simulink model "regs_12B"  (R2018a)
settings: Solver=ode3  StartTime=0.0  StopTime=10.0  FixedStep=.01  RelTol=1e-3  EnableMultiTasking=on
model workspace (MAT data in the model file):
  F = [47.5030304796; 46.9110614304; 47.028984707; 45.6862216169; 44.6182372756; 0]
  FR = [-46.5418915863 -46.5418915863 -46.5418915863 -46.5418915863 -46.5418915863 -46.5418915863 -46.5418915863 -46.5418915863 -46.5418915863 -46.5418915863 -46.5418915863 -46.5418915863 ... (901 elements, 1x901)]
  InputSize = 6
  M = [13.6965475483 27.5033300826 -29.1231309962 -36.2545983973 -28.5352204611 23.5897220685 -14.907640199 1.71607773467 -6.59423100681 35.1253819893 -6.10963272822 7.71481328081 ... (3003 elements, 1001x3)]
  N = 24
  T = table
  T.data = {[13.6965475483 27.5033300826 -29.1231309962 -36.2545983973 -28.5352204611 23.5897220685 -14.907640199 1.71607773467 -6.59423100681 35.1253819893 -6.10963272822 7.71481328081 ... (1001 elements, 1001x1)], [-4.50869960006 8.78080542631 13.3775275088 31.9867982316 4.18537435026 16.5092867395 24.6932352308 2.38519814211 8.8890132209 -4.02964212249 -4.46675798218 1.79304742838 ... (1001 elements, 1001x1)], [-31.9718041188 -26.9402342951 13.2152788717 -38.0977072288 -36.3083467361 23.117797395 10.5331769063 33.1487702757 -5.61173456269 9.59308730026 21.4490888958 -5.45903036842 ... (1001 elements, 1001x1)]}
  T.ndims = 2
  T.nrows = 1001
  T.nvars = 3
  T.varnames = {'Var1', 'Var2', 'Var3'}
  T.props.versionSavedFrom = 2.2
  T.props.minCompatibleVersion = 1
  T.props.incompatibilityMsg = ''
  T.props.VersionSavedFrom = 2.2
  T.props.Description = ''
  T.props.DimensionNames = {'Row', 'Variables'}
  T.props.UserData = []
  T.props.VariableDescriptions = {}
  T.props.VariableUnits = {}
  T.props.VariableContinuity = {}
  X = [0.032483647429 0.400056291337 1.71698946504 0.13508020958 0.621497120838 1.65324546556 1.22373682905 1.82920074721 1.76822087632 0.490626067878 1.91640381392 0.904593399727 1.77711628782 0.929700787381 1.1704427226 0.0233580241983 1.45687078118 0.830600702987 0.237274970231 1.19251283181 0.00937571906531 1.87890955837 1.38282407714 0.543596154356 1.5074746628 1.31666384939 0.567420251723 1.07122901547 0.120432144233 1.35485454959 1.84576620576 0.933277353969]
  a1 = -5.99281334265
  a2 = 6.7586120696
  a3 = -8.48382923723
  axial = 0
  axial_change = [-31.4255261802 -30.7695758416 -31.1885211647 -29.9884626265 -30.6698057294 -31.9546590717 -31.9773114122 -31.0590125801 -31.4973929014 -31.4591407909 -31.9452553476 -31.5912458676 ... (1000 elements, 1000x1)]
  cmd.dt = 0.01
  cmd.transition_v = [0 50 90 1000]
  cmd.transition_y = [0 0 1 1]
  cs : Simulink.ConfigSet (value not decoded)
  curPath = '/Users/khouloud.gaaloul/Documents/Projects/QRA-LocalSearch/Local Search Algorithms/Problems'
  d = 33
  hcvdt_cmd_fcs_dps2 = [0 0 0 0 0 0 0 0 0 0 0 0 ... (1000 elements, 1000x1)]
  height = 0
  height_change = [-31.99975 -31.8 -31.8 -31.8 -31.99975 -31.8 -31.8 -31.8 -31.99975 -31.8 -31.99975 -31.8 ... (1000 elements, 1000x1)]
  hws = Simulink.ModelWorkspace
  i = 7
  j = 16
  lcvdt_cmd_fcs_dps2 = [-172.441967394 -126.914225002 101.408793207 185.523827088 35.8854623366 -8.64188069371 100.038910088 117.411213524 -22.955981386 -181.02871483 29.1905053694 73.1255676915 ... (1000 elements, 1000x1)]
  list(1).name = 'F'
  list(1).size = [6 1]
  list(1).bytes = 48
  list(1).class = 'double'
  list(1).global = 0
  list(1).sparse = 0
  list(1).complex = 0
  list(1).nesting.function = 'simreg'
  list(1).nesting.level = 1
  list(1).persistent = 0
  list(2).name = 'FR'
  list(2).size = [1 901]
  list(2).bytes = 7208
  list(2).class = 'double'
  list(2).global = 0
  list(2).sparse = 0
  list(2).complex = 0
  list(2).nesting.function = 'simreg'
  list(2).nesting.level = 1
  list(2).persistent = 0
  list(3).name = 'InputSize'
  list(3).size = [1 1]
  list(3).bytes = 8
  list(3).class = 'double'
  list(3).global = 0
  list(3).sparse = 0
  list(3).complex = 0
  list(3).nesting.function = 'simreg'
  list(3).nesting.level = 1
  list(3).persistent = 0
  list(4).name = 'N'
  list(4).size = [1 1]
  list(4).bytes = 8
  list(4).class = 'double'
  list(4).global = 0
  list(4).sparse = 0
  list(4).complex = 0
  list(4).nesting.function = 'simreg'
  list(4).nesting.level = 1
  list(4).persistent = 0
  list(5).name = 'X'
  list(5).size = [6 2002]
  list(5).bytes = 96096
  list(5).class = 'double'
  list(5).global = 0
  list(5).sparse = 0
  list(5).complex = 0
  list(5).nesting.function = 'simreg'
  list(5).nesting.level = 1
  list(5).persistent = 0
  list(6).name = 'curPath'
  list(6).size = [1 78]
  list(6).bytes = 156
  list(6).class = 'char'
  list(6).global = 0
  list(6).sparse = 0
  list(6).complex = 0
  list(6).nesting.function = 'simreg'
  list(6).nesting.level = 1
  list(6).persistent = 0
  list(7).name = 'd'
  list(7).size = [1 1]
  list(7).bytes = 8
  list(7).class = 'double'
  list(7).global = 0
  list(7).sparse = 0
  list(7).complex = 0
  list(7).nesting.function = 'simreg'
  list(7).nesting.level = 1
  list(7).persistent = 0
  list(8).name = 'hcvdt_cmd_fcs_dps2'
  list(8).size = [1000 1]
  list(8).bytes = 8000
  list(8).class = 'double'
  list(8).global = 0
  list(8).sparse = 0
  list(8).complex = 0
  list(8).nesting.function = 'simreg'
  list(8).nesting.level = 1
  list(8).persistent = 0
  list(9).name = 'hws'
  list(9).size = [1 1]
  list(9).bytes = 0
  list(9).class = 'Simulink.ModelWorkspace'
  list(9).global = 0
  list(9).sparse = 0
  list(9).complex = 0
  list(9).nesting.function = 'simreg'
  list(9).nesting.level = 1
  list(9).persistent = 0
  list(10).name = 'i'
  list(10).size = [1 1]
  list(10).bytes = 8
  list(10).class = 'double'
  list(10).global = 0
  list(10).sparse = 0
  list(10).complex = 0
  list(10).nesting.function = 'simreg'
  list(10).nesting.level = 1
  list(10).persistent = 0
  list(11).name = 'j'
  list(11).size = [1 1]
  list(11).bytes = 8
  list(11).class = 'double'
  list(11).global = 0
  list(11).sparse = 0
  list(11).complex = 0
  list(11).nesting.function = 'simreg'
  list(11).nesting.level = 1
  list(11).persistent = 0
  list(12).name = 'lcvdt_cmd_fcs_dps2'
  list(12).size = [1000 1]
  list(12).bytes = 8000
  list(12).class = 'double'
  list(12).global = 0
  list(12).sparse = 0
  list(12).complex = 0
  list(12).nesting.function = 'simreg'
  list(12).nesting.level = 1
  list(12).persistent = 0
  list(13).name = 'list'
  list(13).size = [24 1]
  list(13).bytes = 35056
  list(13).class = 'struct'
  list(13).global = 0
  list(13).sparse = 0
  list(13).complex = 0
  list(13).nesting.function = 'simreg'
  list(13).nesting.level = 1
  list(13).persistent = 0
  list(14).name = 'mcvdt_cmd_fcs_dps2'
  list(14).size = [1000 1]
  list(14).bytes = 8000
  list(14).class = 'double'
  list(14).global = 0
  list(14).sparse = 0
  list(14).complex = 0
  list(14).nesting.function = 'simreg'
  list(14).nesting.level = 1
  list(14).persistent = 0
  list(15).name = 'modelpath'
  list(15).size = [1 82]
  list(15).bytes = 164
  list(15).class = 'char'
  list(15).global = 0
  list(15).sparse = 0
  list(15).complex = 0
  list(15).nesting.function = 'simreg'
  list(15).nesting.level = 1
  list(15).persistent = 0
  list(16).name = 'n'
  list(16).size = [1 1]
  list(16).bytes = 8
  list(16).class = 'double'
  list(16).global = 0
  list(16).sparse = 0
  list(16).complex = 0
  list(16).nesting.function = 'simreg'
  list(16).nesting.level = 1
  list(16).persistent = 0
  list(17).name = 'nbrInputs'
  list(17).size = [1 1]
  list(17).bytes = 8
  list(17).class = 'double'
  list(17).global = 0
  list(17).sparse = 0
  list(17).complex = 0
  list(17).nesting.function = 'simreg'
  list(17).nesting.level = 1
  list(17).persistent = 0
  list(18).name = 'nbrTimeSteps'
  list(18).size = [1 1]
  list(18).bytes = 8
  list(18).class = 'double'
  list(18).global = 0
  list(18).sparse = 0
  list(18).complex = 0
  list(18).nesting.function = 'simreg'
  list(18).nesting.level = 1
  list(18).persistent = 0
  list(19).name = 'ncvdt_cmd_fcs_dps2'
  list(19).size = [1000 1]
  list(19).bytes = 8000
  list(19).class = 'double'
  list(19).global = 0
  list(19).sparse = 0
  list(19).complex = 0
  list(19).nesting.function = 'simreg'
  list(19).nesting.level = 1
  list(19).persistent = 0
  list(20).name = 'simOut'
  list(20).size = [1 1]
  list(20).bytes = 54442
  list(20).class = 'Simulink.SimulationOutput'
  list(20).global = 0
  list(20).sparse = 0
  list(20).complex = 0
  list(20).nesting.function = 'simreg'
  list(20).nesting.level = 1
  list(20).persistent = 0
  list(21).name = 't'
  list(21).size = [1 1]
  list(21).bytes = 8
  list(21).class = 'double'
  list(21).global = 0
  list(21).sparse = 0
  list(21).complex = 0
  list(21).nesting.function = 'simreg'
  list(21).nesting.level = 1
  list(21).persistent = 0
  list(22).name = 'var'
  list(22).size = [1 1]
  list(22).bytes = 140328
  list(22).class = 'struct'
  list(22).global = 0
  list(22).sparse = 0
  list(22).complex = 0
  list(22).nesting.function = 'simreg'
  list(22).nesting.level = 1
  list(22).persistent = 0
  list(23).name = 'varout'
  list(23).size = [1000 5]
  list(23).bytes = 40000
  list(23).class = 'double'
  list(23).global = 0
  list(23).sparse = 0
  list(23).complex = 0
  list(23).nesting.function = 'simreg'
  list(23).nesting.level = 1
  list(23).persistent = 0
  list(24).name = 'xcvdt_cmd_fcs_dps2'
  list(24).size = [1000 1]
  list(24).bytes = 8000
  list(24).class = 'double'
  list(24).global = 0
  list(24).sparse = 0
  list(24).complex = 0
  list(24).nesting.function = 'simreg'
  list(24).nesting.level = 1
  list(24).persistent = 0
  mcvdt_cmd_fcs_dps2 = [0 0 0 0 0 0 0 0 0 0 0 0 ... (1000 elements, 1000x1)]
  model_cs : Simulink.ConfigSet (value not decoded)
  modelpath = '/Users/khouloud.gaaloul/Documents/Projects/QRA-LocalSearch/Simulink Models/3_regulators/'
  n = 6
  nbrInputs = 16
  nbrTimeSteps = 1001
  ncvdt_cmd_fcs_dps2 = [0 0 0 0 0 0 0 0 0 0 0 0 ... (1000 elements, 1000x1)]
  pitch = 0
  pitch_change = [-29.1847957495 -33.8637964543 -47.1499761463 -47.1433778125 -41.276337879 -45.6028204159 -37.5507526458 -39.9406146771 -31.3489497461 -28.9458637417 -26.1569554928 -41.8886302088 ... (1000 elements, 1000x1)]
  req = 'R10'
  roll = 0
  roll_change = [-41.4686910833 -44.5265370434 -48.3240218587 -45.9838380142 -45.0248995082 -48.7661309065 -46.4562699575 -48.9496331544 -43.3304519808 -46.1818460958 -48.131234837 -44.5028232735 ... (1000 elements, 1000x1)]
  simOut = Simulink.SimulationOutput
  simOut.Data.tout = [0.01 0.02 0.03 0.04 0.05 0.06 0.07 0.08 0.09 0.1 0.11 0.12 ... (1000 elements, 1000x1)]
  simOut.Data.varout = [-172.441967394 -126.914225002 101.408793207 185.523827088 35.8854623366 -8.64188069371 100.038910088 117.411213524 -22.955981386 -181.02871483 29.1905053694 73.1255676915 ... (5000 elements, 1000x5)]
  simOut.Metadata = Simulink.SimulationMetadata
  simOut.Metadata.ModelInfo.ModelName = 'regs'
  simOut.Metadata.ModelInfo.ModelVersion = '1.40'
  simOut.Metadata.ModelInfo.ModelFilePath = '/Users/khouloud.gaaloul/Documents/Projects/QRA-Search/SimulinkModels/3_regulators/regs.slx'
  simOut.Metadata.ModelInfo.UserID = 'khouloud.gaaloul'
  simOut.Metadata.ModelInfo.MachineName = ''
  simOut.Metadata.ModelInfo.Platform = 'MACI64'
  simOut.Metadata.ModelInfo.ModelStructuralChecksum = [173027761; 2281278173; 3875996436; 2760024160]
  simOut.Metadata.ModelInfo.SimulationMode = 'normal'
  simOut.Metadata.ModelInfo.StartTime = 0
  simOut.Metadata.ModelInfo.StopTime = 10
  simOut.Metadata.ModelInfo.SolverInfo.Type = 'Fixed-Step'
  simOut.Metadata.ModelInfo.SolverInfo.Solver = 'FixedStepDiscrete'
  simOut.Metadata.ModelInfo.SolverInfo.FixedStepSize = 0.01
  simOut.Metadata.ModelInfo.SimulinkVersion.Name = 'Simulink'
  simOut.Metadata.ModelInfo.SimulinkVersion.Version = '8.7'
  simOut.Metadata.ModelInfo.SimulinkVersion.Release = '(R2016a)'
  simOut.Metadata.ModelInfo.SimulinkVersion.Date = '10-Feb-2016'
  simOut.Metadata.TimingInfo.WallClockTimestampStart = '2018-03-19 12:10:18.328231'
  simOut.Metadata.TimingInfo.WallClockTimestampStop = '2018-03-19 12:10:19.216989'
  simOut.Metadata.TimingInfo.InitializationElapsedWallTime = 0.857562
  simOut.Metadata.TimingInfo.ExecutionElapsedWallTime = 0.0059
  simOut.Metadata.TimingInfo.TerminationElapsedWallTime = 0.025314
  simOut.Metadata.TimingInfo.TotalElapsedWallTime = 0.888776
  simOut.Metadata.ExecutionInfo.StopEvent = 'ReachedStopTime'
  simOut.Metadata.ExecutionInfo.StopEventSource = []
  simOut.Metadata.ExecutionInfo.StopEventDescription = 'Reached stop time of 10'
  simOut.Metadata.ExecutionInfo.ErrorDiagnostic = []
  simOut.Metadata.ExecutionInfo.WarningDiagnostics = struct([])
  simOut.Metadata.AppInfo = struct()
  t = [0 0.01 0.02 0.03 0.04 0.05 0.06 0.07 0.08 0.09 0.1 0.11 ... (1001 elements, 1001x1)]
  u = [0.032483647429 0.032483647429 0.032483647429 0.032483647429 0.032483647429 0.032483647429 0.032483647429 0.032483647429 0.032483647429 0.032483647429 0.032483647429 0.032483647429 ... (16016 elements, 1001x16)]
  var.time = [0 0.01 0.02 0.03 0.04 0.05 0.06 0.07 0.08 0.09 0.1 0.11 ... (1001 elements, 1x1001)]
  var.signals(1).values = [0 0 0 0 0 0 0 0 0 0 0 0 ... (1001 elements, 1001x1)]
  var.signals(1).dimensions = 1
  var.signals(2).values = [0 0 0 0 0 0 0 0 0 0 0 0 ... (1001 elements, 1001x1)]
  var.signals(2).dimensions = 1
  var.signals(3).values = [-32.7185675438 -18.5522849548 3.78001601081 15.5815188083 36.1819132054 -17.2231806876 -17.5943876227 -13.0057864031 9.37261247594 -32.1369418892 10.1264127632 10.0220220005 ... (1001 elements, 1001x1)]
  var.signals(3).dimensions = 1
  var.signals(4).values = [0 0 0 0 0 0 0 0 0 0 0 0 ... (1001 elements, 1001x1)]
  var.signals(4).dimensions = 1
  var.signals(5).values = [0 0 0 0 0 0 0 0 0 0 0 0 ... (1001 elements, 1001x1)]
  var.signals(5).dimensions = 1
  var.signals(6).values = [0 0 0 0 0 0 0 0 0 0 0 0 ... (1001 elements, 1001x1)]
  var.signals(6).dimensions = 1
  var.signals(7).values = [0 0 0 0 0 0 0 0 0 0 0 0 ... (1001 elements, 1001x1)]
  var.signals(7).dimensions = 1
  var.signals(8).values = [0 0 0 0 0 0 0 0 0 0 0 0 ... (1001 elements, 1001x1)]
  var.signals(8).dimensions = 1
  var.signals(9).values = [0 0 0 0 0 0 0 0 0 0 0 0 ... (1001 elements, 1001x1)]
  var.signals(9).dimensions = 1
  var.signals(10).values = [0 0 0 0 0 0 0 0 0 0 0 0 ... (1001 elements, 1001x1)]
  var.signals(10).dimensions = 1
  var.signals(11).values = [-29.3225790184 21.8891959243 -11.8121125634 -28.6095603327 30.5189783332 -22.8969150265 17.132242283 30.9103401859 -35.8426218327 -15.1947880413 -18.4250967621 -31.7844478779 ... (1001 elements, 1001x1)]
  var.signals(11).dimensions = 1
  var.signals(12).values = [0 0 0 0 0 0 0 0 0 0 0 0 ... (1001 elements, 1001x1)]
  var.signals(12).dimensions = 1
  var.signals(13).values = [0 0 0 0 0 0 0 0 0 0 0 0 ... (1001 elements, 1001x1)]
  var.signals(13).dimensions = 1
  var.signals(14).values = [0 0 0 0 0 0 0 0 0 0 0 0 ... (1001 elements, 1001x1)]
  var.signals(14).dimensions = 1
  var.signals(15).values = [0 0 0 0 0 0 0 0 0 0 0 0 ... (1001 elements, 1001x1)]
  var.signals(15).dimensions = 1
  var.signals(16).values = [0 0 0 0 0 0 0 0 0 0 0 0 ... (1001 elements, 1001x1)]
  var.signals(16).dimensions = 1
  varout = [-172.441967394 -126.914225002 101.408793207 185.523827088 35.8854623366 -8.64188069371 100.038910088 117.411213524 -22.955981386 -181.02871483 29.1905053694 73.1255676915 ... (5000 elements, 1000x5)]
  vars = {'dt'; 'transition_v'; 'transition_y'}
  xcvdt_cmd_fcs_dps2 = [0 0 0 0 0 0 0 0 0 0 0 0 ... (1000 elements, 1000x1)]
  yaw = 0
  yaw_change = [-49.1533965478 -48.6929062567 -47.6689253182 -47.3940427916 -49.3847503901 -46.8626914945 -44.1531478971 -48.0156975418 -49.8912914581 -49.5126245185 -48.3496741118 -48.8753270352 ... (1000 elements, 1000x1)]
undefined symbols (not defined in the file): dt, transition_v, transition_y
libraries: simulink x2
(part 1 of 2)
settings Model: Creator=elliocm  LastModifiedBy=khouloud.gaaloul
settings DataIOCC: ExternalInput=[t,u]  LimitDataPoints=on  LoadExternalInput=on  SaveFormat=Array  SignalLoggingSaveFormat=ModelDataLogs
settings OptimizationCC: ExpressionDepthLimit=2147483647  LifeSpan=inf
settings DebuggingCC: UnderspecifiedInitializationDetection=Classic  MergeDetectMultiDrivingBlocksExec=none  SolverPrmCheckMsg=warning  FcnCallInpInsideContextMsg=warning  StateNameClashWarn=warning  SFUnexpectedBacktrackingDiag=warning  SFNoUnconditionalDefaultTransitionDiag=warning  SFExecutionAtInitializationDiag=none
settings HardwareCC: ProdBitPerPointer=32  ProdBitPerSizeT=32  ProdBitPerPtrDiffT=32  ProdLargestAtomicFloat=None  ProdIntDivRoundTo=Undefined  ProdEndianess=Unspecified  ProdWordSize=32  ProdHWDeviceType=32-bit Generic
settings ModelReferenceCC: PropagateSignalLabelsOutOfModel=off
settings CodeAppCC: StateflowObjectComments=on
settings GRTTargetCC: TargetLangStandard=C89/C90 (ANSI)  GeneratePreprocessorConditionals=Disable all  CombineOutputUpdateFcns=off  GRTInterface=on
settings ConfigComp: CovMetricSettings=dw  CovHtmlReporting=on  CovSaveCumulativeToWorkspaceVar=on  CovSaveSingleToWorkspaceVar=on  CovExternalEMLEnable=off

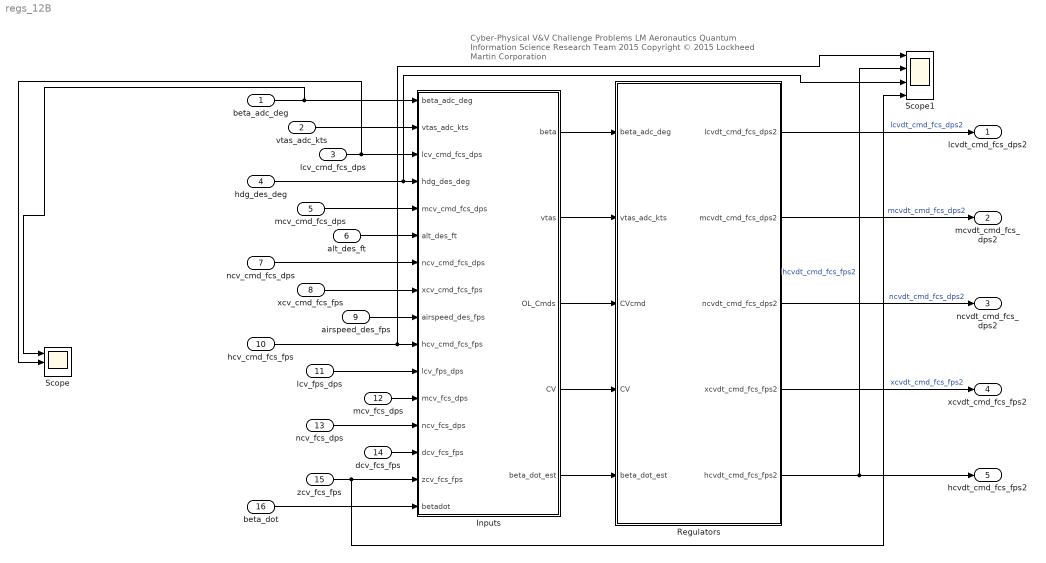
== system regs_12B ==
  note: Cyber-Physical V&V Challenge Problems
      | LM Aeronautics Quantum Information Science Research Team 2015
      | Copyright © 2015 Lockheed Martin Corporation
  beta_adc_deg : Inport  OutDataTypeStr=double
  vtas_adc_kts : Inport  Port=2  OutDataTypeStr=double
  "lcv_cmd_fcs_dps " : Inport  Port=3  OutDataTypeStr=double
  hdg_des_deg : Inport  Port=4  OutDataTypeStr=double
  mcv_cmd_fcs_dps : Inport  Port=5  OutDataTypeStr=double
  alt_des_ft : Inport  Port=6  OutDataTypeStr=double
  ncv_cmd_fcs_dps : Inport  Port=7  OutDataTypeStr=double
  xcv_cmd_fcs_fps : Inport  Port=8  OutDataTypeStr=double
  airspeed_des_fps : Inport  Port=9  OutDataTypeStr=double
  hcv_cmd_fcs_fps : Inport  Port=10  OutDataTypeStr=double
  lcv_fps_dps : Inport  Port=11  OutDataTypeStr=double
  mcv_fcs_dps : Inport  Port=12  OutDataTypeStr=double
  ncv_fcs_dps : Inport  Port=13  OutDataTypeStr=double
  dcv_fcs_fps : Inport  Port=14  OutDataTypeStr=double
  zcv_fcs_fps : Inport  Port=15  OutDataTypeStr=double
  beta_dot : Inport  Port=16  OutDataTypeStr=double
  Inputs : Subsystem
  Regulators : Subsystem
  Scope : Scope  NumInputPorts=3
  Scope1 : Scope  NumInputPorts=4
  lcvdt_cmd_fcs_dps2 : Outport
  mcvdt_cmd_fcs_dps2 : Outport  Port=2
  ncvdt_cmd_fcs_dps2 : Outport  Port=3
  xcvdt_cmd_fcs_fps2 : Outport  Port=4
  hcvdt_cmd_fcs_fps2 : Outport  Port=5
  wires:
  Inputs/4(CV) -> Regulators/4(CV)
  Inputs/3(OL_Cmds) -> Regulators/3(CVcmd)
  Inputs/1(beta) -> Regulators/1(beta_adc_deg)
  Inputs/5(beta_dot_est) -> Regulators/5(beta_dot_est)
  vtas_adc_kts/1 -> Inputs/2(vtas_adc_kts)
  "lcv_cmd_fcs_dps "/1 -> Scope/2, Inputs/3("lcv_cmd_fcs_dps ")
  mcv_cmd_fcs_dps/1 -> Inputs/5(mcv_cmd_fcs_dps)
  ncv_cmd_fcs_dps/1 -> Inputs/7(ncv_cmd_fcs_dps)
  xcv_cmd_fcs_fps/1 -> Inputs/8(xcv_cmd_fcs_fps)
  hcv_cmd_fcs_fps/1 -> Scope1/1, Inputs/10(hcv_cmd_fcs_fps)
  hdg_des_deg/1 -> Scope1/3, Inputs/4(hdg_des_deg)
  alt_des_ft/1 -> Inputs/6(alt_des_ft)
  airspeed_des_fps/1 -> Inputs/9(airspeed_des_fps)
  Regulators/1(lcvdt_cmd_fcs_dps2) -> lcvdt_cmd_fcs_dps2/1  "lcvdt_cmd_fcs_dps2"
  Regulators/2(mcvdt_cmd_fcs_dps2) -> mcvdt_cmd_fcs_dps2/1  "mcvdt_cmd_fcs_dps2"
  Regulators/3(ncvdt_cmd_fcs_dps2) -> ncvdt_cmd_fcs_dps2/1  "ncvdt_cmd_fcs_dps2"
  Regulators/5(hcvdt_cmd_fcs_fps2) -> Scope1/2, hcvdt_cmd_fcs_fps2/1  "hcvdt_cmd_fcs_fps2"
  Regulators/4(xcvdt_cmd_fcs_fps2) -> xcvdt_cmd_fcs_fps2/1  "xcvdt_cmd_fcs_fps2"
  zcv_fcs_fps/1 -> Scope1/4, Inputs/15(zcv_fcs_fps)
  dcv_fcs_fps/1 -> Inputs/14(dcv_fcs_fps)
  lcv_fps_dps/1 -> Inputs/11(lcv_fps_dps)
  mcv_fcs_dps/1 -> Inputs/12(mcv_fcs_dps)
  ncv_fcs_dps/1 -> Inputs/13(ncv_fcs_dps)
  beta_dot/1 -> Inputs/16(betadot)
  Inputs/2(vtas) -> Regulators/2(vtas_adc_kts)
  beta_adc_deg/1 -> Scope/1, Inputs/1(beta_adc_deg)
